simulink model "PID"  (R2025b)
settings: Solver=FixedStepAuto  StartTime=0.0  StopTime=inf  FixedStep=0.01  RelTol=1e-3  EnableMultiTasking=on
undefined symbols (not defined in the file): DiscIntNeverNeededParam, Discrete, dspblkCoreblockFVToolHelper, gcbh, Time
libraries: dspfdesign x6, arduinosensorlib x3, simulink x2, ctrlSharedLib x2, arduinolib x1
settings Model: FPTRunName=Active  SimulationMode=external  ExtModeTrigDuration=2  Creator=ABE  LastModifiedBy=Adham
settings SolverCC: AlgebraicLoopSolver=TrustRegion
settings DataIOCC: LimitDataPoints=on  SaveFormat=Array
settings OptimizationCC: ExpressionDepthLimit=2147483647.0  LifeSpan=Inf  MaxStackSize=64
settings DebuggingCC: UnderspecifiedInitializationDetection=Classic  MergeDetectMultiDrivingBlocksExec=none  FcnCallInpInsideContextMsg=warning  UnconnectedInputMsg=warning  UnconnectedOutputMsg=warning  UnconnectedLineMsg=warning  AllowSymbolicDim=off  StateNameClashWarn=warning  SFUnexpectedBacktrackingDiag=warning  SFNoUnconditionalDefaultTransitionDiag=warning  SFExecutionAtInitializationDiag=none  ArithmeticOperatorsInVariantConditions=warning
settings HardwareCC: ProdBitPerPointer=32.0  ProdBitPerSizeT=32.0  ProdBitPerPtrDiffT=32.0  ProdLargestAtomicInteger=Long  ProdLargestAtomicFloat=Double  ProdWordSize=32.0  ProdHWDeviceType=ARM Compatible->ARM Cortex
settings ModelReferenceCC: EnableRefExpFcnMdlSchedulingChecks=on  PropagateSignalLabelsOutOfModel=off
settings SFSimCC: SimUseLocalCustomCode=off  CustomCodeUndefinedFunction=UseInterfaceOnly
settings RTWCC: SystemTargetFile=ert.tlc  HardwareBoard=ESP32-WROOM (Arduino Compatible)  TemplateMakefile=ert_default_tmf  GenerateReport=on  RTWVerbose=off  RTWUseLocalCustomCode=off  Toolchain=ESP32  BuildConfiguration=Faster Runs  LaunchReport=on  GPUComputeCapability=3.5  Description=Embedded Coder
settings RTWCC: CustomInclude=|
  | C:\ProgramData\MATLAB\SupportPackages\R2025b\aCLI\data\packages\esp32\hardware\esp32\2.0.11\libraries\Wire\src
  | core\inc
  | platform\inc
settings RTWCC: CustomSource=|
  | C:\ProgramData\MATLAB\SupportPackages\R2025b\aCLI\data\packages\esp32\hardware\esp32\2.0.11\libraries\Wire\src\Wire.cpp
  | core\src\vl53l0x_api.cpp
  | core\src\vl53l0x_api_calibration.cpp
  | core\src\vl53l0x_api_core.cpp
  | core\src\vl53l0x_api_ranging.cpp
  | core\src\vl53l0x_api_strings.cpp
  | platform\src\vl53l0x_platform.cpp
  | Adafruit_VL53L0X.cpp
settings CodeAppCC: ForceParamTrailComments=on  OperatorAnnotations=on  StateflowObjectComments=on  MATLABSourceComments=on
settings ERTTargetCC: ExtModeTransport=3.0  ExtModeStaticAlloc=on  ExtModeAutomaticAllocSize=off  ExtModeStaticAllocSize=65536.0  ExtModeMexFile=ext_xcp  ExtModeIntrfLevel=Level2 - Open  InlinedParameterPlacement=Hierarchical  DynamicArrayContainerType=coder::array  MultiwordLength=2048.0  ERTCustomFileBanners=off  SupportContinuousTime=on  SupportNonInlinedSFcns=on  RemoveResetFunc=off  SupportVariableSizeSignals=on  ModelStepFunctionPrototypeControlCompliant=off
settings ConfigComp: CovMetricSettings=dw  CovSaveCumulativeToWorkspaceVar=on  CovSaveSingleToWorkspaceVar=on  CovExternalEMLEnable=off  CovSFcnEnable=off

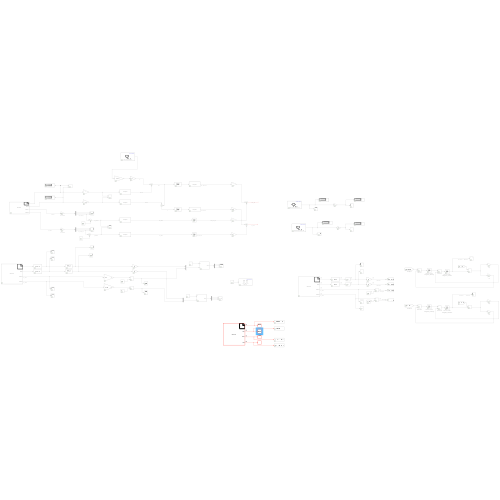
[thumbnail: Simulink's stored preview of the top-level diagram]
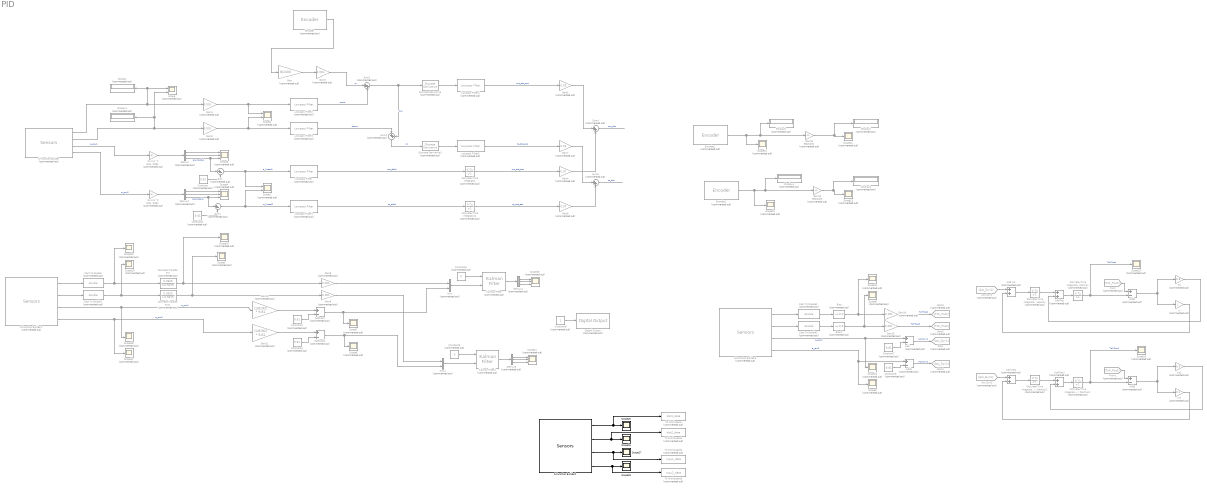
== system PID ==
  Acc Dyn1 : From  Commented=on  GotoTag=Acc_Dyn1
  Acc Dyn2 : From  Commented=on  GotoTag=Acc_Dyn2
  Add{,1..3} (4 alike) : Sum  Commented=on  Inputs=+-
  Add Pos : Sum  Commented=on
  Add Pos2 : Sum  Commented=on
  Add Vel : Sum  Commented=on
  Add Vel2 : Sum  Commented=on
  Bias : Bias  Commented=on  Bias=0.0  SaturateOnIntegerOverflow=off
  Bias1 : Bias  Commented=on  Bias=0.0  SaturateOnIntegerOverflow=off
  Cast To Double{,1..3} (4 alike) : DataTypeConversion  Commented=on  OutDataTypeStr=double  SaturateOnIntegerOverflow=off  RndMeth=Floor
  Constant{,1,3..4,7..8} (6 alike) : Constant  Commented=on  Value=9.81
  Constant2 : Constant  Commented=on  Value=0
  Constant5 : Constant  Commented=on  Value=0
  Constant6 : Constant  Commented=on
  Demux{,1,4..5} (4 alike) : Demux  Commented=on  Outputs=3
  Digital Output : arduinolib/Digital Output  Commented=on  pinNumber=2  Direction=output  blockPlatform=arduino
  Discrete Transfer Fcn : DiscreteTransferFcn  Commented=on  LoadFcn=dspblkCoreblockFVToolHelper(gcbh,'load');  Numerator=[0.0625]  Denominator=[1 -0.9375]
      settings: CopyFcn=dspblkCoreblockFVToolHelper(gcbh,'copy');  DeleteFcn=dspblkCoreblockFVToolHelper(gcbh,'close');  ModelCloseFcn=dspblkCoreblockFVToolHelper(gcbh,'close');  PreSaveFcn=dspblkCoreblockFVToolHelper(gcbh,'presave');  PostSaveFcn=dspblkCoreblockFVToolHelper(gcbh,'postsave');  CloseFcn=dspblkCoreblockFVToolHelper(gcbh,'close');
  Discrete Transfer Fcn1 : DiscreteTransferFcn  Commented=on  LoadFcn=dspblkCoreblockFVToolHelper(gcbh,'load');  Numerator=[0.0625]  Denominator=[1 -0.9375]
      settings: CopyFcn=dspblkCoreblockFVToolHelper(gcbh,'copy');  DeleteFcn=dspblkCoreblockFVToolHelper(gcbh,'close');  ModelCloseFcn=dspblkCoreblockFVToolHelper(gcbh,'close');  PreSaveFcn=dspblkCoreblockFVToolHelper(gcbh,'presave');  PostSaveFcn=dspblkCoreblockFVToolHelper(gcbh,'postsave');  CloseFcn=dspblkCoreblockFVToolHelper(gcbh,'close');
  Discrete Derivative : simulink/Discrete/Discrete Derivative  Commented=on  gainval=1.0  ICPrevScaledInput=0.0  OutMin=[]  OutMax=[]  OutDataType=fixdt(1, 16)  OutScaling=2^-10  DoSatur=off
  Discrete Derivative1 : simulink/Discrete/Discrete Derivative  Commented=on  gainval=1.0  ICPrevScaledInput=0.0  OutMin=[]  OutMax=[]  OutDataType=fixdt(1, 16)  OutScaling=2^-10  DoSatur=off
  Discrete-Time Integrator : DiscreteIntegrator  Commented=on  SampleTime=-1  ICPrevOutput=DiscIntNeverNeededParam  ICPrevScaledInput=DiscIntNeverNeededParam
  Discrete-Time Integrator1 : DiscreteIntegrator  Commented=on  SampleTime=-1  ICPrevOutput=DiscIntNeverNeededParam  ICPrevScaledInput=DiscIntNeverNeededParam
  Discrete-Time Integrator_Position : DiscreteIntegrator  Commented=on  SampleTime=0.04  ICPrevOutput=DiscIntNeverNeededParam  ICPrevScaledInput=DiscIntNeverNeededParam
  Discrete-Time Integrator_Position2 : DiscreteIntegrator  Commented=on  SampleTime=0.04  ICPrevOutput=DiscIntNeverNeededParam  ICPrevScaledInput=DiscIntNeverNeededParam
  Discrete-Time Integrator_Velocity : DiscreteIntegrator  Commented=on  SampleTime=0.04  ICPrevOutput=DiscIntNeverNeededParam  ICPrevScaledInput=DiscIntNeverNeededParam
  Discrete-Time Integrator_Velocity2 : DiscreteIntegrator  Commented=on  SampleTime=0.04  ICPrevOutput=DiscIntNeverNeededParam  ICPrevScaledInput=DiscIntNeverNeededParam
  Display{,1..5} (6 alike) : Display  Commented=on
  Encoder : arduinosensorlib/Encoder  Commented=on  InputA=2  InputB=3  Mode=No reset  SampleTime=-1
  Encoder1 : arduinosensorlib/Encoder  Commented=on  InputA=12  InputB=13  Mode=No reset  SampleTime=-1
  Encoder2 : arduinosensorlib/Encoder  Commented=on  InputA=36  InputB=39  Mode=No reset  SampleTime=-1
  From : From  Commented=on  GotoTag=ToF_Pos1
  From1 : From  Commented=on  GotoTag=ToF_Pos2
  Gain : Gain  Commented=on  Gain=8/2400
  Gain{1..3,8..9,14..15} (7 alike) : Gain  Commented=on  Gain=0.001
  Gain10 : Gain  Commented=on  Gain=(1/8192) * 9.81
  Gain11 : Gain  Commented=on  Gain=(1/8192) * 9.81
  Gain12 : Gain  Commented=on  Gain=360/2400
  Gain13 : Gain  Commented=on  Gain=360/2400
  Gain4 : Gain  Commented=on  Gain=0.97
  Gain5 : Gain  Commented=on  Gain=0.03
  Gain6 : Gain  Commented=on  Gain=0.97
  Gain7 : Gain  Commented=on  Gain=0.03
  Goto : Goto  Commented=on  GotoTag=Acc_Dyn1
  Goto1 : Goto  Commented=on  GotoTag=Acc_Dyn2
  Goto2 : Goto  Commented=on  GotoTag=ToF_Pos2
  Goto3 : Goto  Commented=on  GotoTag=ToF_Pos1
  Kalman Filter : ctrlSharedLib/Kalman Filter  Commented=on  TimeDomain=Discrete-Time  UseCurrentEstimator=on  ModelSource=Individual A, B, C, D matrices  ModelSourceVariable=ss(0.95,1,1,0,1)  A=[1, 0.01, 0.00005; 0, 1, 0.01; 0, 0, 1]  B=[0; 0; 0]  C=[1, 0, 0; 0, 0, 1]  D=[0; 0]  NumberOfStates=1  NumberOfInputs=1  NumberOfOutputs=1  InitialEstimateSource=Dialog  X0=[0; 0; 0]  P0=10  UseK=off  UseGH=off  NumberOfProcessNoiseInputs=1  G=1  TimeInvariantG=on  H=0  TimeInvariantH=on  Q=diag([0.001, 0.01, 0.1])  TimeInvariantQ=on  R=diag([0.01, 0.5])  TimeInvariantR=on  N=0  TimeInvariantN=on  AddInputPort=on  AddEnablePort=off  OutputEstimatedY=off  OutputP=off  Ts=0.01
  Kalman Filter1 : ctrlSharedLib/Kalman Filter  Commented=on  TimeDomain=Discrete-Time  UseCurrentEstimator=on  ModelSource=Individual A, B, C, D matrices  ModelSourceVariable=ss(0.95,1,1,0,1)  A=[1, 0.01, 0.00005; 0, 1, 0.01; 0, 0, 1]  B=[0; 0; 0]  C=[1, 0, 0; 0, 0, 1]  D=[0; 0]  NumberOfStates=1  NumberOfInputs=1  NumberOfOutputs=1  InitialEstimateSource=Dialog  X0=[0; 0; 0]  P0=10  UseK=off  UseGH=off  NumberOfProcessNoiseInputs=1  G=1  TimeInvariantG=on  H=0  TimeInvariantH=on  Q=diag([0.001, 0.01, 0.1])  TimeInvariantQ=on  R=diag([0.01, 0.5])  TimeInvariantR=on  N=0  TimeInvariantN=on  AddInputPort=on  AddEnablePort=off  OutputEstimatedY=off  OutputP=off  Ts=0.01
  Ki : Gain  Commented=on
  Ki2 : Gain  Commented=on  Gain=0.1
  Kp : Gain  Commented=on  Gain=0.8
  Kp2 : Gain  Commented=on  Gain=0.5
  Lowpass Filter : dspfdesign/Lowpass Filter  Commented=on  FilterType=IIR  DesignForMinimumOrder=on  FilterOrder=50  PassbandFrequency=25  StopbandFrequency=40  PassbandRipple=0.5  StopbandAttenuation=40  SampleRateMode=Specify on dialog  SampleRate=200  SimulateUsing=Interpreted execution  roundingMode=Floor  coeffsDataTypeStr=fixdt(1,16)
  Lowpass Filter1 : dspfdesign/Lowpass Filter  Commented=on  FilterType=IIR  DesignForMinimumOrder=on  FilterOrder=50  PassbandFrequency=25  StopbandFrequency=40  PassbandRipple=0.5  StopbandAttenuation=40  SampleRateMode=Specify on dialog  SampleRate=200  SimulateUsing=Interpreted execution  roundingMode=Floor  coeffsDataTypeStr=fixdt(1,16)
  Lowpass Filter2 : dspfdesign/Lowpass Filter  Commented=on  FilterType=IIR  DesignForMinimumOrder=on  FilterOrder=50  PassbandFrequency=8  StopbandFrequency=15  PassbandRipple=0.5  StopbandAttenuation=40  SampleRateMode=Specify on dialog  SampleRate=200  SimulateUsing=Interpreted execution  roundingMode=Floor  coeffsDataTypeStr=fixdt(1,16)
  Lowpass Filter3 : dspfdesign/Lowpass Filter  Commented=on  FilterType=IIR  DesignForMinimumOrder=on  FilterOrder=50  PassbandFrequency=8  StopbandFrequency=15  PassbandRipple=0.5  StopbandAttenuation=40  SampleRateMode=Specify on dialog  SampleRate=200  SimulateUsing=Interpreted execution  roundingMode=Floor  coeffsDataTypeStr=fixdt(1,16)
  Lowpass Filter4 : dspfdesign/Lowpass Filter  Commented=on  FilterType=IIR  DesignForMinimumOrder=on  FilterOrder=50  PassbandFrequency=5  StopbandFrequency=10  PassbandRipple=0.5  StopbandAttenuation=40  SampleRateMode=Specify on dialog  SampleRate=200  SimulateUsing=Interpreted execution  roundingMode=Floor  coeffsDataTypeStr=fixdt(1,16)
  Lowpass Filter5 : dspfdesign/Lowpass Filter  Commented=on  FilterType=IIR  DesignForMinimumOrder=on  FilterOrder=50  PassbandFrequency=5  StopbandFrequency=10  PassbandRipple=0.5  StopbandAttenuation=40  SampleRateMode=Specify on dialog  SampleRate=200  SimulateUsing=Interpreted execution  roundingMode=Floor  coeffsDataTypeStr=fixdt(1,16)
  Mux : Mux  Commented=on  Inputs=2
  Mux1 : Mux  Commented=on  Inputs=2
  S-Function Builder : S-Function  Commented=on  FunctionName=Sensors  SFunctionModules=Sensors_wrapper.cpp  SFunctionDeploymentMode=off  EnableBusSupport=off  mask(S-Function Builder){}
      mask help: Simulink:masks:SFunctionBuilder_MD
      mask init:
      | val = [[.9  0.75 0.75 1 1 .9 .9 1]',[1 1 0.75 0.75 .9 .9 1 .9]'];try , sys = get_param(gcb,'SfunBuilderFcnName');if isempty(sys), sys = get_param(gcb,'FunctionName'); end,catch, sys = get_param(gcb,'FunctionName'); end
      settings: CopyFcn=set_param(gcbh,'LinkStatus','none')  OpenFcn=sfunctionwizard(gcbh)
      mask Display:
      | plot(val(:,1),val(:,2))
      | disp(sys)
      | port_label('output',1,sprintf('%s', 'Dist1'),'interpreter','tex')
      | port_label('output',2,sprintf('%s', 'Dist2'),'interpreter','tex')
      | port_label('output',3,sprintf('%s', 'MPU1'),'interpreter','tex')
      | port_label('output',4,sprintf('%s', 'MPU2'),'interpreter','tex')
  S-Function Builder1 : S-Function  Commented=on  FunctionName=Sensors  SFunctionModules=Sensors_wrapper.cpp  SFunctionDeploymentMode=off  EnableBusSupport=off  mask(S-Function Builder){}
      mask help: Simulink:masks:SFunctionBuilder_MD
      mask init: same as PID/S-Function Builder
      settings: CopyFcn=set_param(gcbh,'LinkStatus','none')  OpenFcn=sfunctionwizard(gcbh)
      mask Display:
      | plot(val(:,1),val(:,2))
      | disp(sys)
      | port_label('output',1,sprintf('%s', 'Dist1'),'interpreter','tex')
      | port_label('output',2,sprintf('%s', 'Dist2'),'interpreter','tex')
      | port_label('output',3,sprintf('%s', 'MPU1'),'interpreter','tex')
      | port_label('output',4,sprintf('%s', 'MPU2'),'interpreter','tex')
  S-Function Builder2 : S-Function  FunctionName=Sensors  SFunctionModules=Sensors_wrapper.cpp  SFunctionDeploymentMode=off  EnableBusSupport=off  mask(S-Function Builder){}
      mask help: Simulink:masks:SFunctionBuilder_MD
      mask init: same as PID/S-Function Builder
      settings: CopyFcn=set_param(gcbh,'LinkStatus','none')  OpenFcn=sfunctionwizard(gcbh)
      mask Display:
      | plot(val(:,1),val(:,2))
      | disp(sys)
      | port_label('output',1,sprintf('%s', 'Pos1'),'interpreter','tex')
      | port_label('output',2,sprintf('%s', 'Vel1'),'interpreter','tex')
      | port_label('output',3,sprintf('%s', 'Pos2'),'interpreter','tex')
      | port_label('output',4,sprintf('%s', 'Vel2'),'interpreter','tex')
  S-Function Builder3 : S-Function  Commented=on  FunctionName=Sensors  SFunctionModules=Sensors_wrapper.cpp  SFunctionDeploymentMode=off  EnableBusSupport=off  mask(S-Function Builder){}
      mask help: Simulink:masks:SFunctionBuilder_MD
      mask init: same as PID/S-Function Builder
      settings: CopyFcn=set_param(gcbh,'LinkStatus','none')  OpenFcn=sfunctionwizard(gcbh)
      mask Display:
      | plot(val(:,1),val(:,2))
      | disp(sys)
      | port_label('output',1,sprintf('%s', 'Dist1'),'interpreter','tex')
      | port_label('output',2,sprintf('%s', 'Dist2'),'interpreter','tex')
      | port_label('output',3,sprintf('%s', 'MPU1'),'interpreter','tex')
      | port_label('output',4,sprintf('%s', 'MPU2'),'interpreter','tex')
  Scope : Scope  Commented=on  NumInputPorts=2
  Scope1 : Scope  Commented=on  NumInputPorts=2
      settings: ActiveDisplayYMinimum=-56.5231010988615  ActiveDisplayYMaximum=12.143746444556918
  Scope{5..15,18..24} (18 alike) : Scope  Commented=on
      Scope10 settings: ActiveDisplayYMinimum=172.5  ActiveDisplayYMaximum=177.5  DataLoggingVariableName=ScopeData10
      Scope11 settings: ActiveDisplayYMinimum=9.744943380355835  ActiveDisplayYMaximum=9.8841536045074463  DataLoggingVariableName=ScopeData11
      Scope12 settings: ActiveDisplayYMinimum=0.050000000023283059  ActiveDisplayYMaximum=0.25000000002328304  DataLoggingVariableName=ScopeData12
      Scope13 settings: ActiveDisplayYMinimum=2.6000000005587935  ActiveDisplayYMaximum=4.6000000005587935  DataLoggingVariableName=ScopeData13
      Scope14 settings: ActiveDisplayYMinimum=0.050000000023283059  ActiveDisplayYMaximum=0.25000000002328304  DataLoggingVariableName=ScopeData14
      Scope15 settings: ActiveDisplayYMinimum=0.050000000023283059  ActiveDisplayYMaximum=0.25000000002328304  DataLoggingVariableName=ScopeData15
      Scope18 settings: ActiveDisplayYMinimum=9.7185419797897339  ActiveDisplayYMaximum=9.863740086555481  DataLoggingVariableName=ScopeData18
      Scope19 settings: ActiveDisplayYMinimum=138.625  ActiveDisplayYMaximum=142.375  DataLoggingVariableName=ScopeData19
      Scope20 settings: ActiveDisplayYMinimum=138.9791157255143  ActiveDisplayYMaximum=142.57285591542686  DataLoggingVariableName=ScopeData5
      Scope21 settings: ActiveDisplayYMinimum=9.7185419797897339  ActiveDisplayYMaximum=9.863740086555481  DataLoggingVariableName=ScopeData8
      Scope22 settings: ActiveDisplayYMinimum=142.5  ActiveDisplayYMaximum=147.5  DataLoggingVariableName=ScopeData9
      Scope23 settings: ActiveDisplayYMinimum=0.071130859344771771  ActiveDisplayYMaximum=0.16145183224733464  DataLoggingVariableName=ScopeData23
      Scope24 settings: ActiveDisplayYMinimum=-0.016486890734338396  ActiveDisplayYMaximum=0.1483820166090456  DataLoggingVariableName=ScopeData24
      Scope5 settings: DataLoggingVariableName=ScopeData20
      Scope6 settings: ActiveDisplayYMinimum=11.203428121805191  ActiveDisplayYMaximum=11.568670781850814  DataLoggingVariableName=ScopeData6
      Scope7 settings: ActiveDisplayYMinimum=12.641073684547115  ActiveDisplayYMaximum=12.909441991397172  DataLoggingVariableName=ScopeData7
      Scope8 settings: ActiveDisplayYMinimum=26.125000000000004  ActiveDisplayYMaximum=194.875  DataLoggingVariableName=ScopeData21
      Scope9 settings: ActiveDisplayYMinimum=9.744943380355835  ActiveDisplayYMaximum=9.8841536045074463  DataLoggingVariableName=ScopeData22
  Scope{3..4,16..17} (4 alike) : Scope  Commented=on  NumInputPorts=3
      Scope16 settings: ActiveDisplayYMinimum=-55.371028048396113  ActiveDisplayYMaximum=7.8369086855649925  DataLoggingVariableName=ScopeData16
      Scope17 settings: ActiveDisplayYMinimum=-55.371028048396113  ActiveDisplayYMaximum=7.8369086855649925  DataLoggingVariableName=ScopeData17
      Scope3 settings: DataLoggingVariableName=ScopeData3
      Scope4 settings: DataLoggingVariableName=ScopeData4
  Scope2 : Scope  Commented=on  NumInputPorts=2
      settings: ActiveDisplayYMinimum=0.48055924091978774  ActiveDisplayYMaximum=0.54691164581733531  DataLoggingVariableName=ScopeData2
  Scope{25..28} (4 alike) : Scope
      Scope25 settings: ActiveDisplayYMinimum=0.12826772220432758  ActiveDisplayYMaximum=0.14402329735457897  DataLoggingVariableName=ScopeData25
      Scope26 settings: ActiveDisplayYMinimum=-0.01661411311943084  ActiveDisplayYMaximum=0.014283073251135647  DataLoggingVariableName=ScopeData26
      Scope27 settings: ActiveDisplayYMinimum=0.14770182967185974  ActiveDisplayYMaximum=0.16801077127456665  DataLoggingVariableName=ScopeData27
      Scope28 settings: ActiveDisplayYMinimum=-0.02719685051124543  ActiveDisplayYMaximum=0.019924065913073719  DataLoggingVariableName=ScopeData28
  Subtract : Sum  Commented=on  Inputs=+-
  Subtract1 : Sum  Commented=on  Inputs=+-
  Sum : Sum  Commented=on  Inputs=|+-
  Sum1 : Sum  Commented=on  Inputs=|+-
  Sum{2..5} (4 alike) : Sum  Commented=on  Inputs=|++
  To Workspace : ToWorkspace  Commented=on  VariableName=dist1_data  SaveFormat=Timeseries  SampleTime=-1
  To Workspace1 : ToWorkspace  Commented=on  VariableName=dist2_data  SaveFormat=Timeseries  SampleTime=-1
  To Workspace2 : ToWorkspace  Commented=on  VariableName=mpu1_data  SaveFormat=Timeseries  SampleTime=-1
  To Workspace3 : ToWorkspace  Commented=on  VariableName=mpu2_data  SaveFormat=Timeseries  SampleTime=-1
  To m/s^2 : Gain  Commented=on  Gain=9.81 / 8192
  to m/s^2 : Gain  Commented=on  Gain=9.81 / 8192
  wires:
  S-Function Builder/3 -> To m/s^2/1  "a_raw1"
  Demux/1 -> Scope3/1
  Demux/2 -> Scope3/2
  Demux/3 -> Sum/1, Scope3/3  "az_mps2_1"
  Demux1/2 -> Scope4/2
  Demux1/1 -> Scope4/1
  S-Function Builder/4 -> to m/s^2/1  "a_raw2"
  To m/s^2/1 -> Demux/1
  to m/s^2/1 -> Demux1/1
  S-Function Builder/1 -> Scope/1, Display/1, Gain1/1
  S-Function Builder/2 -> Scope/2, Display1/1, Gain2/1
  Constant/1 -> Sum/2
  Sum/1 -> Lowpass Filter/1, Scope1/1  "a_linear1"
  Sum1/1 -> Lowpass Filter1/1, Scope1/2  "a_linear2"
  Constant1/1 -> Sum1/2
  Demux1/3 -> Sum1/1, Scope4/3  "az_mps2_2"
  Gain1/1 -> Scope2/1, Lowpass Filter2/1
  Gain2/1 -> Scope2/2, Lowpass Filter3/1
  Encoder/1 -> Gain/1
  Gain/1 -> Gain3/1
  Lowpass Filter2/1 -> Sum2/2  "zus-zr"
  Lowpass Filter3/1 -> Sum3/1  "zs-zus"
  Lowpass Filter/1 -> Discrete-Time Integrator/1  "zus_ddot"
  Lowpass Filter1/1 -> Discrete-Time Integrator1/1  "zs_ddot"
  Sum2/1 -> Discrete Derivative/1, Sum3/2  "zus"
  Gain3/1 -> Sum2/1  "zr"
  Discrete Derivative/1 -> Lowpass Filter4/1
  Lowpass Filter4/1 -> Gain5/1  "zus_dot_pos"
  Lowpass Filter5/1 -> Gain7/1  "zs_dot_pos"
  Discrete Derivative1/1 -> Lowpass Filter5/1
  Sum3/1 -> Discrete Derivative1/1  "zs"
  Discrete-Time Integrator/1 -> Gain4/1  "zus_dot_acc"
  Discrete-Time Integrator1/1 -> Gain6/1  "zs_dot_acc"
  Gain5/1 -> Sum4/1
  Gain4/1 -> Sum4/2
  Sum4/1 -> ?  "zus_dot"
  Gain7/1 -> Sum5/1
  Gain6/1 -> Sum5/2
  Sum5/1 -> ?  "zs_dot"
  Constant2/1 -> Kalman Filter/1
  S-Function Builder1/3 -> Gain10/1, Scope18/1  "a_raw1"
  S-Function Builder1/4 -> Gain11/1, Scope11/1  "a_raw2"
  Gain10/1 -> Subtract/1
  Gain11/1 -> Subtract1/1
  Constant3/1 -> Subtract/2
  Constant4/1 -> Subtract1/2
  Gain8/1 -> Mux/1
  Subtract/1 -> Mux/2, Scope7/1
  Mux/1 -> Kalman Filter/2
  Kalman Filter/1 -> Demux4/1
  Kalman Filter1/1 -> Demux5/1
  Mux1/1 -> Kalman Filter1/2
  Subtract1/1 -> Mux1/2, Scope6/1
  Gain9/1 -> Mux1/1
  Constant5/1 -> Kalman Filter1/1
  S-Function Builder1/1 -> Cast To Double/1
  S-Function Builder1/2 -> Cast To Double1/1
  Constant6/1 -> Digital Output/1
  Encoder2/1 -> Scope15/1, Display4/1, Gain13/1
  Encoder1/1 -> Scope14/1, Display5/1, Gain12/1
  Gain12/1 -> Display2/1, Scope12/1
  Gain13/1 -> Scope13/1, Display3/1
  Demux4/1 -> Scope16/1
  Demux4/2 -> Scope16/2
  Demux4/3 -> Scope16/3
  Demux5/1 -> Scope17/1
  Demux5/2 -> Scope17/2
  Demux5/3 -> Scope17/3
  Cast To Double/1 -> Scope19/1, Discrete Transfer Fcn/1
  Cast To Double1/1 -> Scope10/1, Discrete Transfer Fcn1/1
  Discrete Transfer Fcn1/1 -> Scope5/1, Gain9/1
  Discrete Transfer Fcn/1 -> Scope20/1, Gain8/1
  Cast To Double3/1 -> Bias1/1
  Cast To Double2/1 -> Bias/1
  S-Function Builder3/2 -> Cast To Double3/1
  S-Function Builder3/4 -> Add1/1, Scope9/1  "a_raw2"
  S-Function Builder3/3 -> Scope21/1, Add/1  "a_raw1"
  Constant7/1 -> Add/2
  Constant8/1 -> Add1/2
  Gain14/1 -> Goto3/1  "ToF Pos1"
  Gain15/1 -> Goto2/1  "ToF Pos2"
  Add/1 -> Goto/1  "Acc Dyn1"
  Add1/1 -> Goto1/1  "Acc Dyn2"
  Acc Dyn1/1 -> Add Vel/1
  Add Vel/1 -> Discrete-Time Integrator_Velocity/1
  Discrete-Time Integrator_Velocity/1 -> Add Pos/1
  Add Pos/1 -> Discrete-Time Integrator_Position/1
  From/1 -> Add2/1
  Add2/1 -> Ki/1, Kp/1
  Add3/1 -> Kp2/1, Ki2/1
  From1/1 -> Add3/1
  Add Pos2/1 -> Discrete-Time Integrator_Position2/1
  Discrete-Time Integrator_Velocity2/1 -> Add Pos2/1
  Add Vel2/1 -> Discrete-Time Integrator_Velocity2/1
  Acc Dyn2/1 -> Add Vel2/1
  Kp/1 -> Add Pos/2
  Ki/1 -> Add Vel/2
  Kp2/1 -> Add Pos2/2
  Ki2/1 -> Add Vel2/2
  Discrete-Time Integrator_Position/1 -> Scope23/1, Add2/2  "ToF Pos1"
  Discrete-Time Integrator_Position2/1 -> Scope24/1, Add3/2  "ToF Pos1"
  Bias/1 -> Gain14/1, Scope22/1
  Bias1/1 -> Gain15/1, Scope8/1
  S-Function Builder3/1 -> Cast To Double2/1
  S-Function Builder2/4 -> To Workspace3/1, Scope28/1
  S-Function Builder2/3 -> To Workspace2/1, Scope27/1
  S-Function Builder2/2 -> To Workspace1/1, Scope26/1
  S-Function Builder2/1 -> To Workspace/1, Scope25/1
